simulink model "scalar"  (R2021a)
settings: Solver=ode1  StartTime=0.0001  StopTime=25  FixedStep=.001  RelTol=1e-3
model workspace (MAT data in the model file):
  T = Simulink.Parameter
  T.Value = 0
  T.DataType = 'auto'
  T.Min = 0
  T.Max = 100
  T.Dimensions = [1 1]
settings Model: Creator=RUDRA  LastModifiedBy=RUDRA

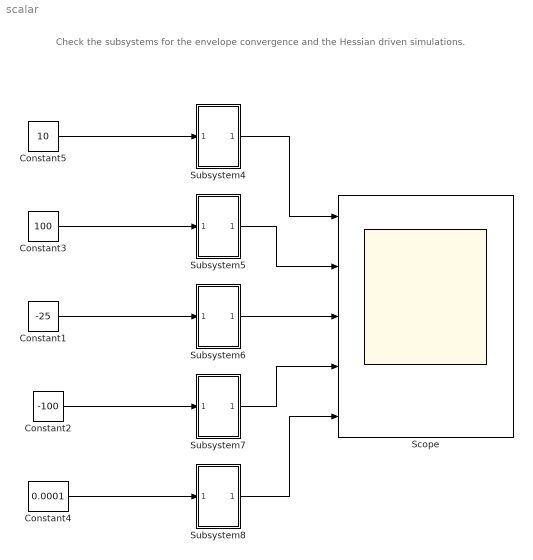
== system scalar ==
  note: Check the subsystems for the envelope convergence and the Hessian driven simulations.
  Constant1 : Constant  Value=-25
  Constant2 : Constant  Value=-100
  Constant3 : Constant  Value=100
  Constant4 : Constant  Value=0.0001
  Constant5 : Constant  Value=10
  Scope : Scope  NumInputPorts=5
  Subsystem4 : Subsystem
  Subsystem5 : Subsystem
  Subsystem6 : Subsystem
  Subsystem7 : Subsystem
  Subsystem8 : Subsystem
  wires:
  Constant3/1 -> Subsystem5/1(In1)
  Constant1/1 -> Subsystem6/1(In1)
  Constant2/1 -> Subsystem7/1(In1)
  Constant4/1 -> Subsystem8/1(In1)
  Constant5/1 -> Subsystem4/1(In1)
  Subsystem4/1(Output1) -> Scope/1
  Subsystem5/1(Output1) -> Scope/2
  Subsystem6/1(Output1) -> Scope/3
  Subsystem7/1(Output1) -> Scope/4
  Subsystem8/1(Output1) -> Scope/5

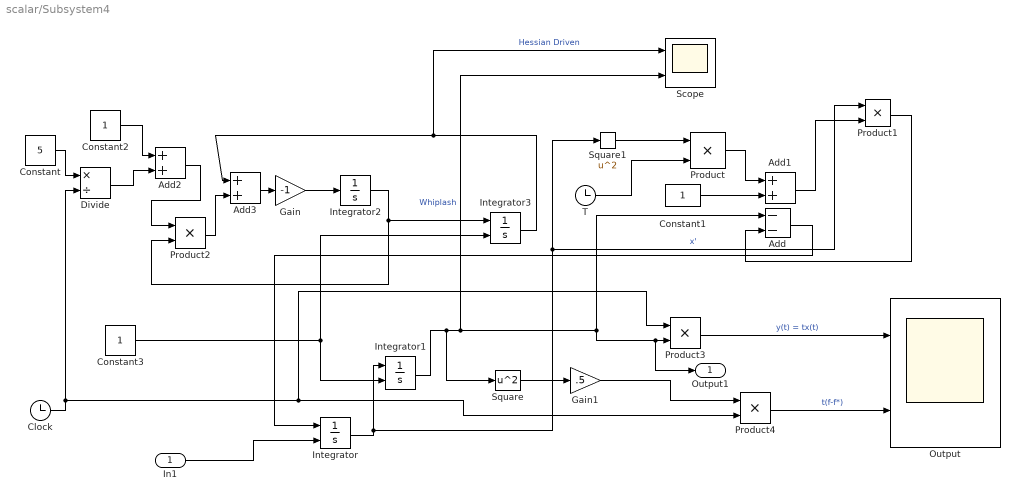
== system scalar/Subsystem4 ==
  In1 : Inport
  Add : Sum  Inputs=--
  Add1 : Sum
  Add2 : Sum
  Add3 : Sum
  Clock : Clock
  Constant : Constant  Value=5
  Constant1 : Constant
  Constant2 : Constant
  Constant3 : Constant
  Divide : Product  Inputs=*/
  Gain : Gain  Gain=-1
  Gain1 : Gain  Gain=.5
  Integrator : Integrator  InitialConditionSource=external
  Integrator1 : Integrator  InitialConditionSource=external  InitialCondition=5
  Integrator2 : Integrator
  Integrator3 : Integrator  InitialConditionSource=external  InitialCondition=5
  Output : Scope  NumInputPorts=2
  Product{,1..4} (5 alike) : Product
  Scope : Scope  NumInputPorts=2
  Square : Math  Operator=square  SaturateOnIntegerOverflow=on
  Square1 : Math  Operator=square  SaturateOnIntegerOverflow=on
  T : Clock
  Output1 : Outport
  wires:
  Integrator/1 -> Square1/1, Product1/1, Integrator1/1  "x'"
  Integrator1/1 -> Scope/2, Output1/1, Product3/2, Add/1, Square/1  "Whiplash"
  Add2/1 -> Product2/1
  Add1/1 -> Product1/2
  Constant/1 -> Divide/1
  Square/1 -> Gain1/1
  Product1/1 -> Add/2
  Integrator3/1 -> Add3/1, Scope/1  "Hessian Driven"
  Product4/1 -> Output/2  "t(f-f*)"
  Add3/1 -> Gain/1
  Product/1 -> Add1/1
  Add/1 -> Integrator/1
  Gain/1 -> Integrator2/1
  Square1/1 -> Product/1
  Clock/1 -> Divide/2, Product4/2, Product3/1
  Divide/1 -> Add2/2
  Constant1/1 -> Add1/2
  Product2/1 -> Add3/2
  Constant3/1 -> Integrator1/2, Integrator3/2
  Product3/1 -> Output/1  "y(t) = tx(t)"
  Constant2/1 -> Add2/1
  T/1 -> Product/2
  Integrator2/1 -> Product2/2, Integrator3/1
  Gain1/1 -> Product4/1
  In1/1 -> Integrator/2

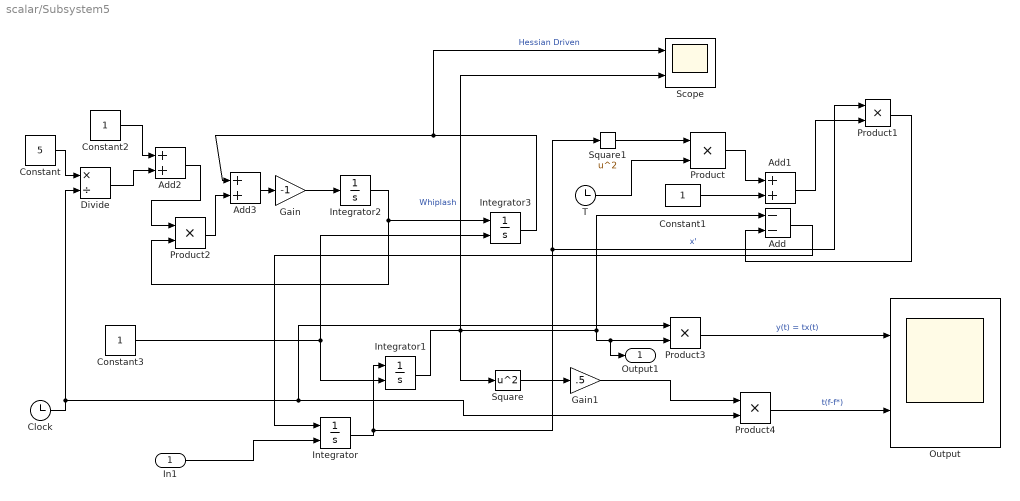
== system scalar/Subsystem5 ==
  In1 : Inport
  Add : Sum  Inputs=--
  Add1 : Sum
  Add2 : Sum
  Add3 : Sum
  Clock : Clock
  Constant : Constant  Value=5
  Constant1 : Constant
  Constant2 : Constant
  Constant3 : Constant
  Divide : Product  Inputs=*/
  Gain : Gain  Gain=-1
  Gain1 : Gain  Gain=.5
  Integrator : Integrator  InitialConditionSource=external
  Integrator1 : Integrator  InitialConditionSource=external  InitialCondition=5
  Integrator2 : Integrator
  Integrator3 : Integrator  InitialConditionSource=external  InitialCondition=5
  Output : Scope  NumInputPorts=2
  Product{,1..4} (5 alike) : Product
  Scope : Scope  NumInputPorts=2
  Square : Math  Operator=square  SaturateOnIntegerOverflow=on
  Square1 : Math  Operator=square  SaturateOnIntegerOverflow=on
  T : Clock
  Output1 : Outport
  wires:
  Integrator/1 -> Square1/1, Product1/1, Integrator1/1  "x'"
  Integrator1/1 -> Scope/2, Output1/1, Product3/2, Add/1, Square/1  "Whiplash"
  Add2/1 -> Product2/1
  Add1/1 -> Product1/2
  Constant/1 -> Divide/1
  Square/1 -> Gain1/1
  Product1/1 -> Add/2
  Integrator3/1 -> Add3/1, Scope/1  "Hessian Driven"
  Product4/1 -> Output/2  "t(f-f*)"
  Add3/1 -> Gain/1
  Product/1 -> Add1/1
  Add/1 -> Integrator/1
  Gain/1 -> Integrator2/1
  Square1/1 -> Product/1
  Clock/1 -> Divide/2, Product4/2, Product3/1
  Divide/1 -> Add2/2
  Constant1/1 -> Add1/2
  Product2/1 -> Add3/2
  Constant3/1 -> Integrator1/2, Integrator3/2
  Product3/1 -> Output/1  "y(t) = tx(t)"
  Constant2/1 -> Add2/1
  T/1 -> Product/2
  Integrator2/1 -> Product2/2, Integrator3/1
  Gain1/1 -> Product4/1
  In1/1 -> Integrator/2

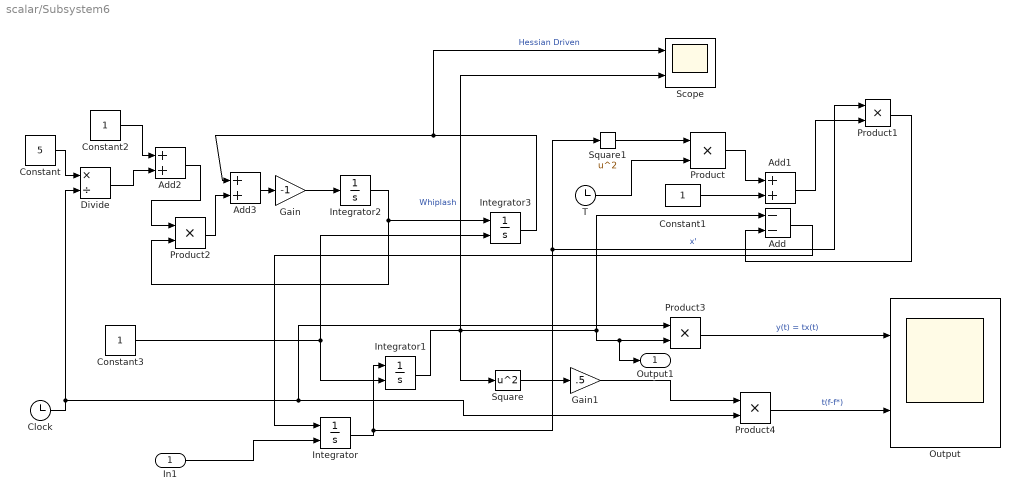
== system scalar/Subsystem6 ==
  In1 : Inport
  Add : Sum  Inputs=--
  Add1 : Sum
  Add2 : Sum
  Add3 : Sum
  Clock : Clock
  Constant : Constant  Value=5
  Constant1 : Constant
  Constant2 : Constant
  Constant3 : Constant
  Divide : Product  Inputs=*/
  Gain : Gain  Gain=-1
  Gain1 : Gain  Gain=.5
  Integrator : Integrator  InitialConditionSource=external
  Integrator1 : Integrator  InitialConditionSource=external  InitialCondition=5
  Integrator2 : Integrator
  Integrator3 : Integrator  InitialConditionSource=external  InitialCondition=5
  Output : Scope  NumInputPorts=2
  Product{,1..4} (5 alike) : Product
  Scope : Scope  NumInputPorts=2
  Square : Math  Operator=square  SaturateOnIntegerOverflow=on
  Square1 : Math  Operator=square  SaturateOnIntegerOverflow=on
  T : Clock
  Output1 : Outport
  wires:
  Integrator/1 -> Square1/1, Product1/1, Integrator1/1  "x'"
  Integrator1/1 -> Scope/2, Output1/1, Product3/2, Add/1, Square/1  "Whiplash"
  Add2/1 -> Product2/1
  Add1/1 -> Product1/2
  Constant/1 -> Divide/1
  Square/1 -> Gain1/1
  Product1/1 -> Add/2
  Integrator3/1 -> Add3/1, Scope/1  "Hessian Driven"
  Product4/1 -> Output/2  "t(f-f*)"
  Add3/1 -> Gain/1
  Product/1 -> Add1/1
  Add/1 -> Integrator/1
  Gain/1 -> Integrator2/1
  Square1/1 -> Product/1
  Clock/1 -> Divide/2, Product4/2, Product3/1
  Divide/1 -> Add2/2
  Constant1/1 -> Add1/2
  Product2/1 -> Add3/2
  Constant3/1 -> Integrator1/2, Integrator3/2
  Product3/1 -> Output/1  "y(t) = tx(t)"
  Constant2/1 -> Add2/1
  T/1 -> Product/2
  Integrator2/1 -> Product2/2, Integrator3/1
  Gain1/1 -> Product4/1
  In1/1 -> Integrator/2

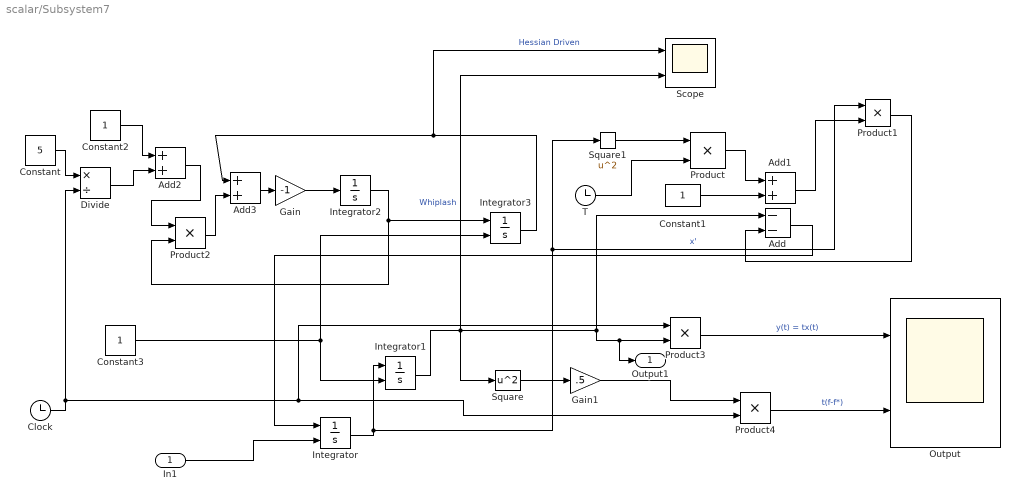
== system scalar/Subsystem7 ==
  In1 : Inport
  Add : Sum  Inputs=--
  Add1 : Sum
  Add2 : Sum
  Add3 : Sum
  Clock : Clock
  Constant : Constant  Value=5
  Constant1 : Constant
  Constant2 : Constant
  Constant3 : Constant
  Divide : Product  Inputs=*/
  Gain : Gain  Gain=-1
  Gain1 : Gain  Gain=.5
  Integrator : Integrator  InitialConditionSource=external
  Integrator1 : Integrator  InitialConditionSource=external  InitialCondition=5
  Integrator2 : Integrator
  Integrator3 : Integrator  InitialConditionSource=external  InitialCondition=5
  Output : Scope  NumInputPorts=2
  Product{,1..4} (5 alike) : Product
  Scope : Scope  NumInputPorts=2
  Square : Math  Operator=square  SaturateOnIntegerOverflow=on
  Square1 : Math  Operator=square  SaturateOnIntegerOverflow=on
  T : Clock
  Output1 : Outport
  wires:
  Integrator/1 -> Square1/1, Product1/1, Integrator1/1  "x'"
  Integrator1/1 -> Scope/2, Output1/1, Product3/2, Add/1, Square/1  "Whiplash"
  Add2/1 -> Product2/1
  Add1/1 -> Product1/2
  Constant/1 -> Divide/1
  Square/1 -> Gain1/1
  Product1/1 -> Add/2
  Integrator3/1 -> Add3/1, Scope/1  "Hessian Driven"
  Product4/1 -> Output/2  "t(f-f*)"
  Add3/1 -> Gain/1
  Product/1 -> Add1/1
  Add/1 -> Integrator/1
  Gain/1 -> Integrator2/1
  Square1/1 -> Product/1
  Clock/1 -> Divide/2, Product4/2, Product3/1
  Divide/1 -> Add2/2
  Constant1/1 -> Add1/2
  Product2/1 -> Add3/2
  Constant3/1 -> Integrator1/2, Integrator3/2
  Product3/1 -> Output/1  "y(t) = tx(t)"
  Constant2/1 -> Add2/1
  T/1 -> Product/2
  Integrator2/1 -> Product2/2, Integrator3/1
  Gain1/1 -> Product4/1
  In1/1 -> Integrator/2

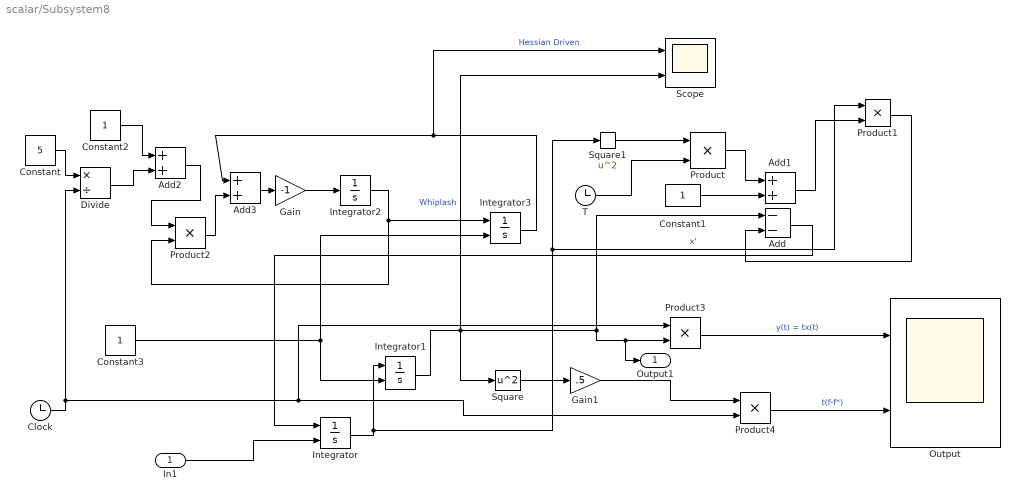
== system scalar/Subsystem8 ==
  In1 : Inport
  Add : Sum  Inputs=--
  Add1 : Sum
  Add2 : Sum
  Add3 : Sum
  Clock : Clock
  Constant : Constant  Value=5
  Constant1 : Constant
  Constant2 : Constant
  Constant3 : Constant
  Divide : Product  Inputs=*/
  Gain : Gain  Gain=-1
  Gain1 : Gain  Gain=.5
  Integrator : Integrator  InitialConditionSource=external
  Integrator1 : Integrator  InitialConditionSource=external  InitialCondition=5
  Integrator2 : Integrator
  Integrator3 : Integrator  InitialConditionSource=external  InitialCondition=5
  Output : Scope  NumInputPorts=2
  Product{,1..4} (5 alike) : Product
  Scope : Scope  NumInputPorts=2
  Square : Math  Operator=square  SaturateOnIntegerOverflow=on
  Square1 : Math  Operator=square  SaturateOnIntegerOverflow=on
  T : Clock
  Output1 : Outport
  wires:
  Integrator/1 -> Square1/1, Product1/1, Integrator1/1  "x'"
  Integrator1/1 -> Scope/2, Output1/1, Product3/2, Add/1, Square/1  "Whiplash"
  Add2/1 -> Product2/1
  Add1/1 -> Product1/2
  Constant/1 -> Divide/1
  Square/1 -> Gain1/1
  Product1/1 -> Add/2
  Integrator3/1 -> Add3/1, Scope/1  "Hessian Driven"
  Product4/1 -> Output/2  "t(f-f*)"
  Add3/1 -> Gain/1
  Product/1 -> Add1/1
  Add/1 -> Integrator/1
  Gain/1 -> Integrator2/1
  Square1/1 -> Product/1
  Clock/1 -> Divide/2, Product4/2, Product3/1
  Divide/1 -> Add2/2
  Constant1/1 -> Add1/2
  Product2/1 -> Add3/2
  Constant3/1 -> Integrator1/2, Integrator3/2
  Product3/1 -> Output/1  "y(t) = tx(t)"
  Constant2/1 -> Add2/1
  T/1 -> Product/2
  Integrator2/1 -> Product2/2, Integrator3/1
  Gain1/1 -> Product4/1
  In1/1 -> Integrator/2
